simulink model "Intermedio_1"  (R2023b)
settings: Solver=VariableStepAuto  StartTime=0.0  StopTime=10.0  RelTol=1e-3
values from neighbouring files (symbols this model uses):
  g = 9.81    [Inizializzazione_Simulink_linearizzazione.m]    (also in inizializzazione_carroponte.m; inizializzazione_carroponte_controllo.m; inizializzazione_carroponte_controllo_ok.m)
undefined symbols (not defined in the file or in its folder): cs, ks, ku, Ls, Lu, ms, mu
settings Model: Creator=drhou  LastModifiedBy=drhou

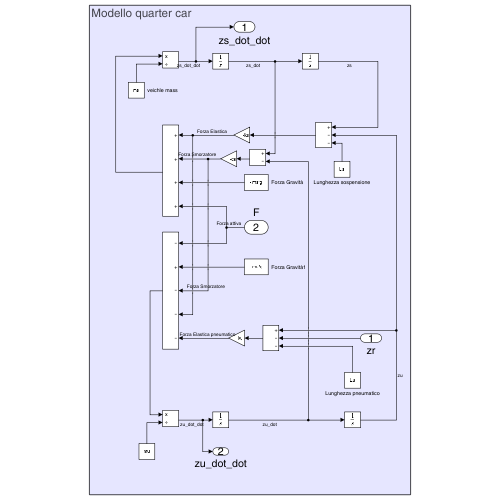
[thumbnail: Simulink's stored preview of the top-level diagram]
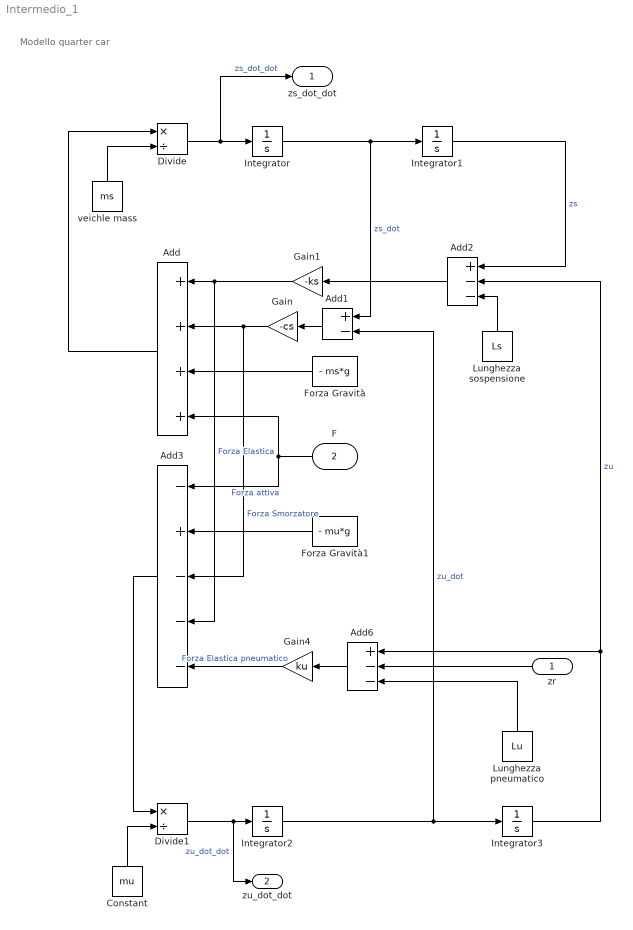
== system Intermedio_1 ==
  note: Modello quarter car
  zr : Inport
  F : Inport  Port=2
  Add : Sum  Inputs=++++
  Add1 : Sum  Inputs=+-
  Add2 : Sum  Inputs=+--
  Add3 : Sum  Inputs=-+---
  Add6 : Sum  Inputs=+--
  Constant : Constant  Value=mu
  Divide : Product  Inputs=*/
  Divide1 : Product  Inputs=*/
  Forza Gravità : Constant  Value=- ms*g
  Forza Gravità1 : Constant  Value=- mu*g
  Gain : Gain  Gain=-cs
  Gain1 : Gain  Gain=-ks
  Gain4 : Gain  Gain=ku
  Integrator{,1..3} (4 alike) : Integrator
  Lunghezza pneumatico : Constant  Value=Lu
  Lunghezza sospensione : Constant  Value=Ls
  veichle mass : Constant  Value=ms
  zs_dot_dot : Outport
  zu_dot_dot : Outport  Port=2
  wires:
  Lunghezza pneumatico/1 -> Add6/3
  Forza Gravità/1 -> Add/3
  Add6/1 -> Gain4/1
  Forza Gravità1/1 -> Add3/2
  Constant/1 -> Divide1/2
  zr/1 -> Add6/2
  Divide/1 -> zs_dot_dot/1, Integrator/1  "zs_dot_dot"
  Gain4/1 -> Add3/5  "Forza Elastica pneumatico"
  Integrator/1 -> Integrator1/1, Add1/1  "zs_dot"
  Add/1 -> Divide/1
  Divide1/1 -> zu_dot_dot/1, Integrator2/1  "zu_dot_dot"
  Integrator2/1 -> Integrator3/1, Add1/2  "zu_dot"
  veichle mass/1 -> Divide/2
  Add3/1 -> Divide1/1
  Add2/1 -> Gain1/1
  Integrator1/1 -> Add2/1  "zs"
  Add1/1 -> Gain/1
  Integrator3/1 -> Add6/1, Add2/2  "zu"
  Gain/1 -> Add/2, Add3/3  "Forza Smorzatore"
  Lunghezza sospensione/1 -> Add2/3
  Gain1/1 -> Add3/4, Add/1  "Forza Elastica"
  F/1 -> Add/4, Add3/1  "Forza attiva"
